simulink model "nlmodel"  (R2020a)
settings: Solver=FixedStepAuto  StartTime=0.0  StopTime=U1(end,1)  RelTol=1e-3
values from neighbouring files (symbols this model uses):
  alpha1hat = 0.0114    [Linearize_whitebox.m]    (also in Linearize_whitebox_final.m; lqr_whitebox.mat; matrices.mat)
  alpha2hat = 0.0079    [Linearize_whitebox.m]    (also in Linearize_whitebox_final.m; lqr_whitebox.mat; matrices.mat)
  area = 0.001    [nonlinid.m]
  area_s = 0.0002    [nonlinid.m]
  boltz = 5.67e-8    (= 5.67e-08)    [Linearize_whitebox.m]    (also in Linearize_whitebox_final.m; lqr_whitebox.mat; matrices.mat; nonlinid.m)
  cphat = 501.9208    [Linearize_whitebox.m]    (also in Linearize_whitebox_final.m; lqr_whitebox.mat; matrices.mat)
  emis = 0.9    [nonlinid.m]
  h = tout(2)-tout(1)    [Linearize_whitebox.m]    (also in Linearize_whitebox_final.m; Observer_mat.m; lqr_whitebox.mat = 1.00037043897; matrices.mat = 1.00080032013)
  m = 0.0052    [model.m]    (also in nonlinid.m = 0.004)
  Tamb = 18+273    (= 291)    [nonlinid.m]
  tau = 24.4408    [model.m]    (also in nonlinid.m = 24)
  uhat = 10.2021    [Linearize_whitebox.m]    (also in Linearize_whitebox_final.m; lqr_whitebox.mat; matrices.mat)
  ushat = 13.8985    [Linearize_whitebox.m]    (also in Linearize_whitebox_final.m; lqr_whitebox.mat; matrices.mat)
  x0 = [y1(1);y2(1)]    [Linearize_whitebox.m]    (also in Linearize_whitebox_final.m; lqr_whitebox.mat = [0 0]; matrices.mat = [293.042473118 292.064956012]; nonlinid.m)
settings Model: Creator=Eveline  LastModifiedBy=Eveline
settings DataIOCC: ReturnWorkspaceOutputs=off  StateSaveName=xm  TimeSaveName=tm
settings DebuggingCC: AlgebraicLoopMsg=none  ArtificialAlgebraicLoopMsg=none  ModelReferenceExtraNoncontSigs=none  OperatingPointInterfaceChecksumMismatchMsg=none

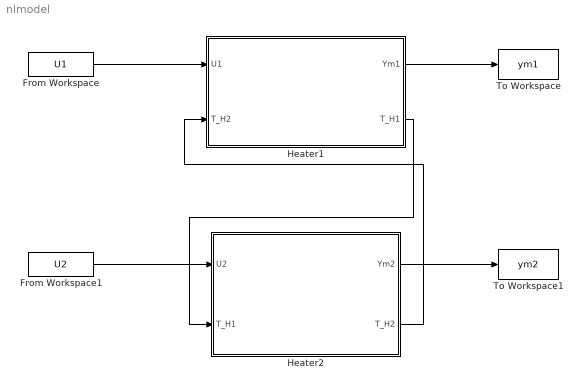
== system nlmodel ==
  From Workspace : FromWorkspace  VariableName=U1  SampleTime=h
  From Workspace1 : FromWorkspace  VariableName=U2  SampleTime=h
  Heater1 : Subsystem
  Heater2 : Subsystem
  To Workspace : ToWorkspace  VariableName=ym1  SampleTime=h
  To Workspace1 : ToWorkspace  VariableName=ym2  SampleTime=h
  wires:
  From Workspace/1 -> Heater1/1(U1)
  Heater1/1(Ym1) -> To Workspace/1
  From Workspace1/1 -> Heater2/1(U2)
  Heater1/2(T_H1) -> Heater2/2(T_H1)
  Heater2/2(T_H2) -> Heater1/2(T_H2)
  Heater2/1(Ym2) -> To Workspace1/1

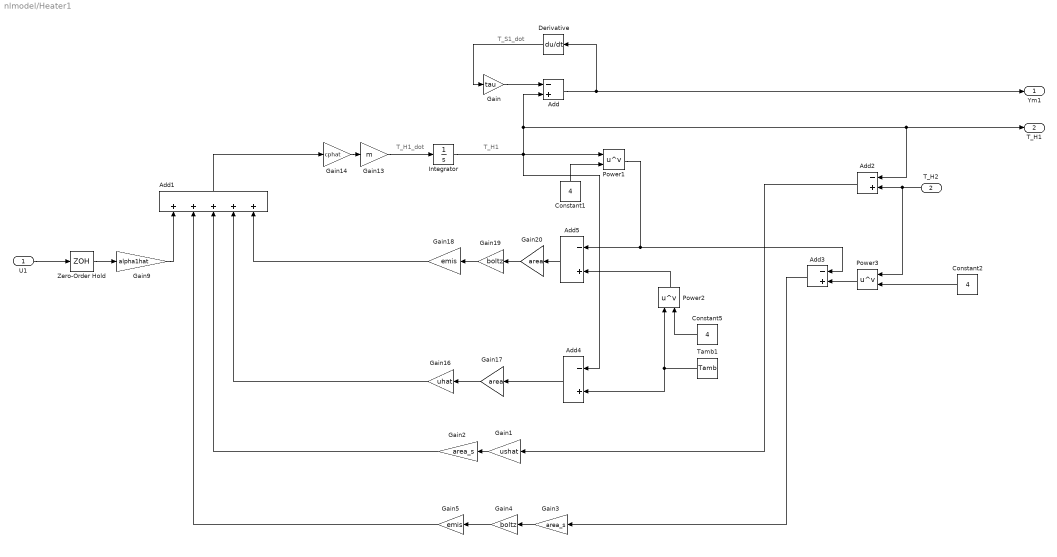
== system nlmodel/Heater1 ==
  note: T_S1_dot
  note: T_H1
  note: T_H1_dot
  U1 : Inport
  T_H2 : Inport  Port=2
  Add{,2..5} (5 alike) : Sum  Inputs=-+
  Add1 : Sum  Inputs=+++++
  Constant1 : Constant  Value=4
  Constant2 : Constant  Value=4
  Constant5 : Constant  Value=4
  Derivative : Derivative
  Gain : Gain  Gain=tau
  Gain1 : Gain  Gain=ushat
  Gain13 : Gain  Gain=m
  Gain14 : Gain  Gain=cphat
  Gain16 : Gain  Gain=uhat
  Gain17 : Gain  Gain=area
  Gain18 : Gain  Gain=emis
  Gain19 : Gain  Gain=boltz
  Gain2 : Gain  Gain=area_s
  Gain20 : Gain  Gain=area
  Gain3 : Gain  Gain=area_s
  Gain4 : Gain  Gain=boltz
  Gain5 : Gain  Gain=emis
  Gain9 : Gain  Gain=alpha1hat
  Integrator : Integrator  InitialCondition=x0(1)
  Power1 : Math  Operator=pow  SaturateOnIntegerOverflow=on
  Power2 : Math  Operator=pow  SaturateOnIntegerOverflow=on
  Power3 : Math  Operator=pow  SaturateOnIntegerOverflow=on
  Tamb1 : Constant  Value=Tamb
  Zero-Order Hold : ZeroOrderHold  SampleTime=-1
  Ym1 : Outport
  T_H1 : Outport  Port=2
  wires:
  Add/1 -> Ym1/1, Derivative/1
  Gain17/1 -> Gain16/1
  Constant5/1 -> Power2/2
  Integrator/1 -> Add4/1, Add2/1, T_H1/1, Add/2, Power1/1
  Constant1/1 -> Power1/2
  Derivative/1 -> Gain/1
  Gain14/1 -> Gain13/1
  Add5/1 -> Gain20/1
  Add1/1 -> Gain14/1
  Add4/1 -> Gain17/1
  Gain20/1 -> Gain19/1
  Tamb1/1 -> Add4/2, Power2/1
  Gain13/1 -> Integrator/1
  Power2/1 -> Add5/2
  Power1/1 -> Add3/1, Add5/1
  Gain/1 -> Add/1
  Gain19/1 -> Gain18/1
  Gain18/1 -> Add1/5
  Gain9/1 -> Add1/1
  Gain16/1 -> Add1/4
  Gain1/1 -> Gain2/1
  T_H2/1 -> Power3/1, Add2/2
  Add2/1 -> Gain1/1
  Gain2/1 -> Add1/3
  Constant2/1 -> Power3/2
  Power3/1 -> Add3/2
  Gain4/1 -> Gain5/1
  Gain3/1 -> Gain4/1
  Add3/1 -> Gain3/1
  Gain5/1 -> Add1/2
  U1/1 -> Zero-Order Hold/1
  Zero-Order Hold/1 -> Gain9/1

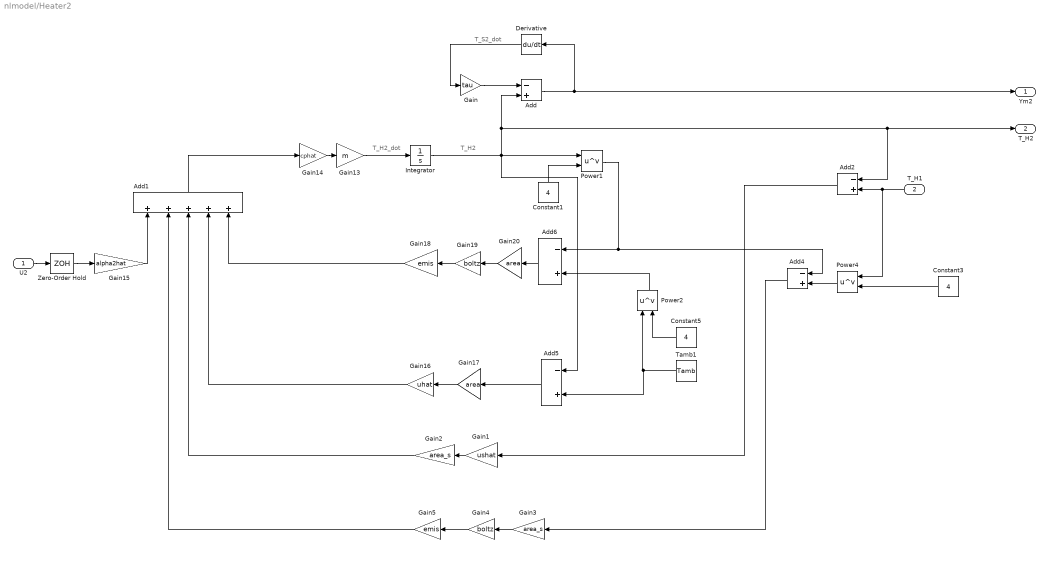
== system nlmodel/Heater2 ==
  note: T_H2
  note: T_H2_dot
  note: T_S2_dot
  U2 : Inport
  T_H1 : Inport  Port=2
  Add{,2,4..6} (5 alike) : Sum  Inputs=-+
  Add1 : Sum  Inputs=+++++
  Constant1 : Constant  Value=4
  Constant3 : Constant  Value=4
  Constant5 : Constant  Value=4
  Derivative : Derivative
  Gain : Gain  Gain=tau
  Gain1 : Gain  Gain=ushat
  Gain13 : Gain  Gain=m
  Gain14 : Gain  Gain=cphat
  Gain15 : Gain  Gain=alpha2hat
  Gain16 : Gain  Gain=uhat
  Gain17 : Gain  Gain=area
  Gain18 : Gain  Gain=emis
  Gain19 : Gain  Gain=boltz
  Gain2 : Gain  Gain=area_s
  Gain20 : Gain  Gain=area
  Gain3 : Gain  Gain=area_s
  Gain4 : Gain  Gain=boltz
  Gain5 : Gain  Gain=emis
  Integrator : Integrator  InitialCondition=x0(2)
  Power1 : Math  Operator=pow  SaturateOnIntegerOverflow=on
  Power2 : Math  Operator=pow  SaturateOnIntegerOverflow=on
  Power4 : Math  Operator=pow  SaturateOnIntegerOverflow=on
  Tamb1 : Constant  Value=Tamb
  Zero-Order Hold : ZeroOrderHold  SampleTime=-1
  Ym2 : Outport
  T_H2 : Outport  Port=2
  wires:
  Gain17/1 -> Gain16/1
  Power4/1 -> Add4/2
  Gain20/1 -> Gain19/1
  Tamb1/1 -> Add5/2, Power2/1
  Constant3/1 -> Power4/2
  Power1/1 -> Add4/1, Add6/1
  Integrator/1 -> Add5/1, T_H2/1, Add2/1, Add/2, Power1/1
  Gain/1 -> Add/1
  Add6/1 -> Gain20/1
  Gain14/1 -> Gain13/1
  Gain1/1 -> Gain2/1
  Add4/1 -> Gain3/1
  Gain18/1 -> Add1/5
  Power2/1 -> Add6/2
  Add/1 -> Ym2/1, Derivative/1
  Gain4/1 -> Gain5/1
  Derivative/1 -> Gain/1
  Constant1/1 -> Power1/2
  Add2/1 -> Gain1/1
  Constant5/1 -> Power2/2
  Add5/1 -> Gain17/1
  Add1/1 -> Gain14/1
  Gain2/1 -> Add1/3
  Gain5/1 -> Add1/2
  T_H1/1 -> Power4/1, Add2/2
  Gain13/1 -> Integrator/1
  Gain19/1 -> Gain18/1
  Gain16/1 -> Add1/4
  Gain3/1 -> Gain4/1
  Gain15/1 -> Add1/1
  U2/1 -> Zero-Order Hold/1
  Zero-Order Hold/1 -> Gain15/1
